simulink model "brain"  (Simulink 7.5)
settings: Solver=FixedStepDiscrete  StartTime=0.0  StopTime=inf  FixedStep=0.2  RelTol=1e-3
values from neighbouring files (symbols this model uses):
  Buoy1_Hue = 0.4    [brainconstants.m]    (also in brainconstants_David.m = 30)
  Buoy1_Saturation = 1.0    (= 1)    [brainconstants.m]    (also in brainconstants_David.m)
  Buoy1_Value = 0.45    [brainconstants.m]    (also in brainconstants_David.m)
  Buoy2_Hue = 0.0    (= 0)    [brainconstants.m]    (also in brainconstants_David.m = 80)
  Buoy2_Saturation = 1.0    (= 1)    [brainconstants.m]    (also in brainconstants_David.m)
  Buoy2_Value = 0.75    [brainconstants.m]    (also in brainconstants_David.m)
  Buoy_Max_Eccentricity = 0.7    [brainconstants.m]    (also in brainconstants_David.m = 1.2)
  Buoy_Max_Extent = 0.9    [brainconstants.m]    (also in brainconstants_David.m)
  Buoy_Min_Eccentricity = 0    [brainconstants.m]    (also in brainconstants_David.m)
  Buoy_Min_Extent = 0.7    [brainconstants.m]    (also in brainconstants_David.m = 0.1)
  Buoy_Strafe = 40    [brainconstants.m]    (also in brainconstants_David.m)
  Cam_Down_Strafe_XPos_Kd = 0.0    (= 0)    [brainconstants.m]    (also in brainconstants_David.m)
  Cam_Down_Strafe_XPos_Ki = 0.0    (= 0)    [brainconstants.m]    (also in brainconstants_David.m)
  Cam_Down_Strafe_XPos_Kp = -1.0    (= -1)    [brainconstants.m]    (also in brainconstants_David.m)
  Cam_Down_Yaw_XPos_Kd = 0.0    (= 0)    [brainconstants.m]    (also in brainconstants_David.m)
  Cam_Down_Yaw_XPos_Ki = 0.0    (= 0)    [brainconstants.m]    (also in brainconstants_David.m)
  Cam_Down_Yaw_XPos_Kp = 0.6    [brainconstants.m]    (also in brainconstants_David.m)
  Cam_Down_YPos_Kd = 0.0    (= 0)    [brainconstants.m]    (also in brainconstants_David.m)
  Cam_Down_YPos_Ki = 0.0    (= 0)    [brainconstants.m]    (also in brainconstants_David.m)
  Cam_Down_YPos_Kp = 0.75    [brainconstants.m]    (also in brainconstants_David.m)
  Cam_Forward_XPosition_Kd = 0.0    (= 0)    [brainconstants.m]    (also in brainconstants_David.m)
  Cam_Forward_XPosition_Ki = 0.0    (= 0)    [brainconstants.m]    (also in brainconstants_David.m)
  Cam_Forward_XPosition_Kp = 0.07    [brainconstants.m]    (also in brainconstants_David.m)
  Cam_Forward_YPosition_Kd = 0.0    (= 0)    [brainconstants.m]    (also in brainconstants_David.m)
  Cam_Forward_YPosition_Ki = 0.0    (= 0)    [brainconstants.m]    (also in brainconstants_David.m)
  Cam_Forward_YPosition_Kp = 0.8    [brainconstants.m]    (also in brainconstants_David.m)
  Depth_Kd = 0.0    (= 0)    [brainconstants.m]    (also in brainconstants_David.m)
  Depth_Ki = 0.0    (= 0)    [brainconstants.m]    (also in brainconstants_David.m)
  Depth_Kp = 75    [brainconstants.m]    (also in brainconstants_David.m)
  Heading_Forward_Velocity = 30    [brainconstants.m]    (also in brainconstants_David.m)
  Heading_Kd = 0.4    [brainconstants.m]    (also in brainconstants_David.m)
  Heading_Ki = 0.0    (= 0)    [brainconstants.m]    (also in brainconstants_David.m)
  Heading_Kp = 0.65    [brainconstants.m]    (also in brainconstants_David.m)
  Hedge_Hue = .4    (= 0.4)    [brainconstants.m]    (also in brainconstants_David.m)
  Hedge_Saturation = 1    [brainconstants.m]    (also in brainconstants_David.m)
  Hedge_Value = .75    (= 0.75)    [brainconstants.m]    (also in brainconstants_David.m)
  Iter_Segment_Thresh = 60    [brainconstants.m]    (also in brainconstants_David.m)
  MissionPlan = [1 1 1 1 1 1 1 1 1 1 1 1 1 0 0 0 0 0 0 0]    [brainconstants.m]    (also in brainconstants_David.m)
  Track_Desired_Depth = 8    [brainconstants.m]    (also in brainconstants_David.m)
  Track_HueHigher = 0.75    [brainconstants.m]    (also in brainconstants_David.m)
  Track_HueLower = 0.4    [brainconstants.m]    (also in brainconstants_David.m)
  Track_Min_Eccentricity = 0.9    [brainconstants.m]    (also in brainconstants_David.m)
  Track_Saturation = 0.75    [brainconstants.m]    (also in brainconstants_David.m)
  Vision_Forward_Velocity = 15    [brainconstants.m]    (also in brainconstants_David.m)
undefined symbols (not defined in the file or in its folder): DiscIntNeverNeededParam, gray, Rec, SDTV, strel, YawRate_Kd, YawRate_Ki, YawRate_Kp
libraries: vipconversions x32, simulink x26, vipgeotforms x9, vipstatistics x9, viptextngfix x7, vipmorphops x6, viptransforms x4, vipsnks x3, vipsrcs x1
(part 6 of 6)

== matlab function StateFlow Functions/StateFlowFunctions.JumpHedge.IterativeSegmentation/Segmentation/Reference Color Selection ==
  data: L input double; ref_colors output double; a input double; b input double; num_colors output double; Dist_Thresh input double
function [ref_colors, num_colors] = Segmentation(L,a,b,Dist_Thresh)
% This function tries segmentation by adding new reference colors everytime
% a pixel is found with a distance greater than a certain amount from
% every other reference color

[rows cols] = size(L);

Dist_Threshold = Dist_Thresh;% L = 0 to 100, a = -100 to 100, b = -100 to 100
                    % max dist = 300 -> 60/300 is 20%
x = 1;  % coefficients determining distance calculation
y = 1.5;
z = 1.5;

max_num_colors = 50;
ref_colors = zeros(max_num_colors,3);   % At most 50 different reference colors
LabelMatrix = zeros(rows,cols);
num_colors = 1;

center_row = floor(rows/2);
center_col = floor(cols/2);

ref_colors(1,:) = [L(center_row,center_col) a(center_row,center_col) b(center_row,center_col)];

flag = 0;
i = 1;
j = 1;
while(i <= rows)        % perform initial segmentation
    while(i <= rows && flag == 0)
        while(j <= cols && flag == 0)
            k = 1;
            min_dist = 1000;
            index = 1;
            while(k <= num_colors)
                dist = sqrt(x*(ref_colors(k,1) - L(i,j))^2 + y*(ref_colors(k,2) - a(i,j))^2 + z*(ref_colors(k,3) - b(i,j))^2);
                if(min_dist > dist)
                    min_dist = double(dist);
                    index = k;
                end
                k = k + 1;
            end
            if(j == 117)
                cow = 1;
            end
            if(min_dist > Dist_Threshold && num_colors < max_num_colors)
                ref_colors(num_colors+1,:) = [L(i,j) a(i,j) b(i,j)];
                num_colors = num_colors + 1;
                flag = 1;
                i = 0;
                j = 0;
            else
                LabelMatrix(i,j) = index;
            end
            j = j + 1;
        end
        j = 1;
        i = i + 1;
    end
    flag = 0;
end

% Go through image once more to get more accurate values for the different regions
ref_color_L_avg = zeros(50,1);
ref_color_a_avg = zeros(50,1);
ref_color_b_avg = zeros(50,1);
color_count = zeros(50,1);
for i = 1:rows
    for j = 1:cols
        index = LabelMatrix(i,j);
        ref_color_L_avg(index) = ref_color_L_avg(index) + L(i,j);
        ref_color_a_avg(index) = ref_color_a_avg(index) + a(i,j);
        ref_color_b_avg(index) = ref_color_b_avg(index) + b(i,j);
        color_count(index) = color_count(index) + 1;
    end
end
ref_color_L_avg = ref_color_L_avg ./ color_count;
ref_color_a_avg = ref_color_a_avg ./ color_count;
ref_color_b_avg = ref_color_b_avg ./ color_count;

for i = 1:num_colors
    ref_colors(i,1) = ref_color_L_avg(i);
    ref_colors(i,2) = ref_color_a_avg(i);
    ref_colors(i,3) = ref_color_b_avg(i);
end

return

== matlab function StateFlow Functions/StateManagement.Running.Autonomous.Perform/Checking to see if state will be performed ==
  data: State1 input double; Done1 output double; MissionPlan input double
function Done1 = CheckPlan(State1,MissionPlan)
% This function checks to see if the current state should be executed

if(MissionPlan(State1) ~= 0)
    Done1 = 0;
else
    Done1 = 1;
end

return

== matlab function StateFlow Functions/StateFlowFunctions.FollowOnePath.OnePath.CamDown_CenterOver_Yaw/Embedded MATLAB Function ==
  data: Area1 input double; Centroid1 input double; BlobCentroidX output double; BlobCentroidY output double; Image input double
function [BlobCentroidX, BlobCentroidY] = PickBiggestBlob(Area1, Centroid1, Image)
% This function will choose and return data about the largest blob given a 
% set of blobs

if(Centroid1(1,1) == -1 && Centroid1(2,1) == -1)
    [ImageY ImageX] = size(Image);
    BlobCentroidX = floor(ImageX/2);
    BlobCentroidY = floor(ImageY/2);
    BlobArea = -1;
else
    [BlobArea, index] = max(double(Area1));
    BlobCentroidX = Centroid1(2, index);
    BlobCentroidY = Centroid1(1, index);
end

return

== matlab function StateFlow Functions/StateFlowFunctions.FollowOnePath.OnePath.CamDown_CenterOver_Yaw/Embedded MATLAB Function1 ==
  data: Image input double; XCenter output double; YCenter output double
function [XCenter,YCenter] = GetImageCenter(Image)
% This function finds the center of an image

[rows cols] = size(Image);

XCenter = floor(cols/2);
YCenter = floor(rows/2);

return
